simulink model "ex11"  (R2023b)
settings: Solver=VariableStepAuto  StartTime=0.0  StopTime=10.0  RelTol=1e-3
settings Model: Creator=sorin  LastModifiedBy=sorin

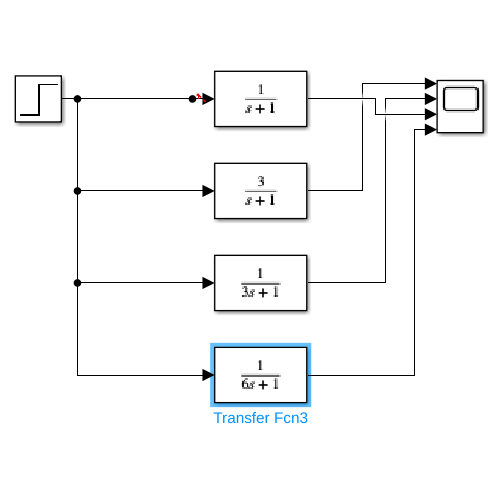
[thumbnail: Simulink's stored preview of the top-level diagram]
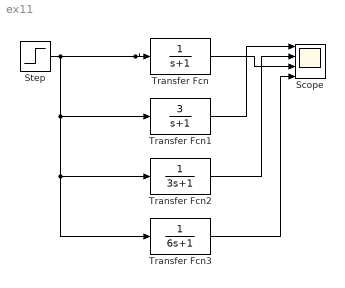
== system ex11 ==
  Scope : Scope  NumInputPorts=4
  Step : Step  SampleTime=0
  Transfer Fcn : TransferFcn  Denominator=[1 1]
  Transfer Fcn1 : TransferFcn  Numerator=[3]  Denominator=[1 1]
  Transfer Fcn2 : TransferFcn  Denominator=[3 1]
  Transfer Fcn3 : TransferFcn  Denominator=[6 1]
  wires:
  Transfer Fcn/1 -> Scope/3
  Transfer Fcn1/1 -> Scope/1
  Step/1 -> Transfer Fcn3/1, Transfer Fcn2/1, Transfer Fcn1/1, Transfer Fcn/1
  Transfer Fcn2/1 -> Scope/2
  Transfer Fcn3/1 -> Scope/4
